simulink model "linear_model"  (R2016b)
settings: Solver=VariableStepAuto  StartTime=0.0  StopTime=10.0  RelTol=1e-3
libraries: simulink x3
settings Model: Creator=sxh  LastModifiedBy=sxh

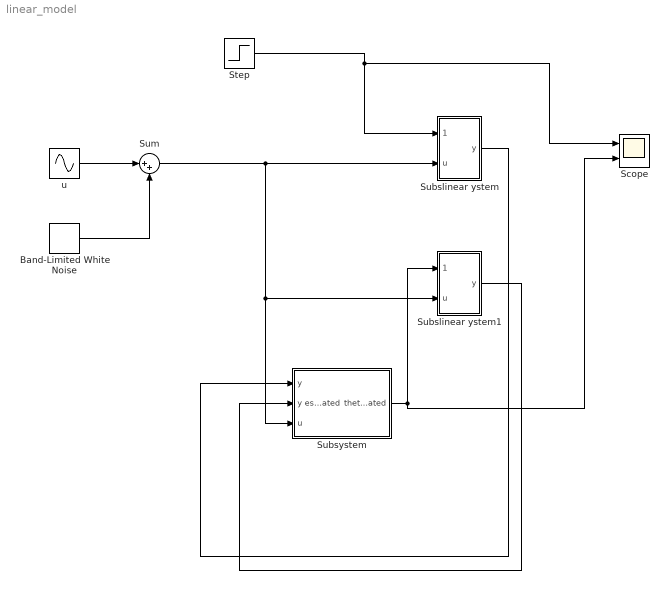
== system linear_model ==
  Band-Limited White Noise : simulink/Sources/Band-Limited White Noise  Cov=0.001  Ts=0.1  seed=[23341]
  Scope : Scope  NumInputPorts=2
  Step : Step  Time=5  Before=1  After=2  SampleTime=0
  Subslinear ystem : Subsystem
  Subslinear ystem1 : Subsystem
  Subsystem : Subsystem
  Sum : Sum  Inputs=|++
  u : Sin  Amplitude=10  SampleTime=0
  wires:
  u/1 -> Sum/1
  Band-Limited White Noise/1 -> Sum/2
  Sum/1 -> Subslinear ystem/2(u), Subslinear ystem1/2(u), Subsystem/3(u)
  Step/1 -> Scope/1, Subslinear ystem/1(theta)
  Subsystem/1(theta estimated) -> Scope/2, Subslinear ystem1/1(theta)
  Subslinear ystem/1(y) -> Subsystem/1(y)
  Subslinear ystem1/1(y) -> Subsystem/2(y estimated)

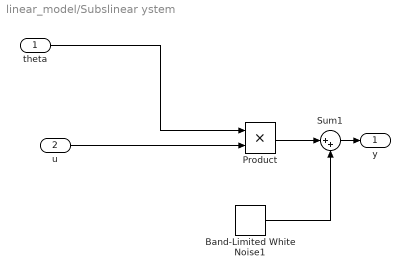
== system linear_model/Subslinear ystem ==
  theta : Inport
  u : Inport  Port=2
  Band-Limited White Noise1 : simulink/Sources/Band-Limited White Noise  Cov=0.1  Ts=0.1  seed=[23341]
  Product : Product
  Sum1 : Sum  Inputs=|++
  y : Outport
  wires:
  u/1 -> Product/2
  Product/1 -> Sum1/1
  theta/1 -> Product/1
  Band-Limited White Noise1/1 -> Sum1/2
  Sum1/1 -> y/1

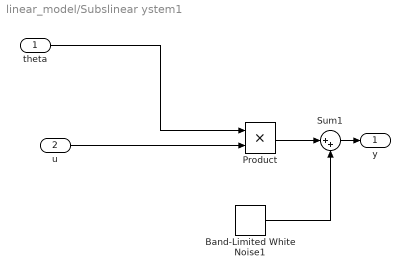
== system linear_model/Subslinear ystem1 ==
  theta : Inport
  u : Inport  Port=2
  Band-Limited White Noise1 : simulink/Sources/Band-Limited White Noise  Cov=0.1  Ts=0.1  seed=[23341]
  Product : Product
  Sum1 : Sum  Inputs=|++
  y : Outport
  wires:
  u/1 -> Product/2
  Product/1 -> Sum1/1
  theta/1 -> Product/1
  Band-Limited White Noise1/1 -> Sum1/2
  Sum1/1 -> y/1

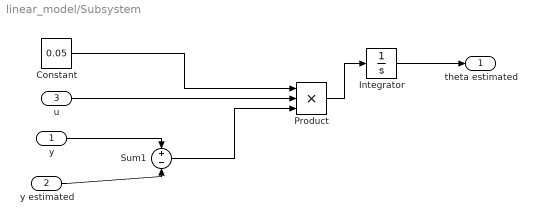
== system linear_model/Subsystem ==
  y : Inport
  y estimated : Inport  Port=2
  u : Inport  Port=3
  Constant : Constant  Value=0.05
  Integrator : Integrator
  Product : Product  Inputs=3
  Sum1 : Sum  Inputs=+-
  theta estimated : Outport
  wires:
  y estimated/1 -> Sum1/2
  Sum1/1 -> Product/3
  y/1 -> Sum1/1
  Constant/1 -> Product/1
  Integrator/1 -> theta estimated/1
  Product/1 -> Integrator/1
  u/1 -> Product/2
